simulink model "HydroEye_6DOF_SITL"  (R2024b)
settings: Solver=VariableStepAuto  StartTime=0.0  StopTime=1200  RelTol=1e-3
values from neighbouring files (symbols this model uses):
  b = 2    [HydroEye.m]
  c = 0.35    [HydroEye.m]
  CD = reshape(AeroLong.CD,length(alpha),length(elevator))    [HydroEye.m]
  cg = [0.5808 0 0.01]    [HydroEye.m]
  CL = reshape(AeroLong.CL,length(alpha),length(elevator))    [HydroEye.m]
  Cl = reshape(AeroLat.Cl,length(beta),length(rudder))    [HydroEye.m]
  Clp = -0.46415*pi/180    (= -0.00810094572313)    [HydroEye.m]
  Clr = 0.12437*pi/180    (= 0.00217066599071)    [HydroEye.m]
  Cm = reshape(AeroLong.Cm,length(alpha),length(elevator))    [HydroEye.m]
  Cmq = -5.4623*pi/180    (= -0.0953351197317)    [HydroEye.m]
  Cn = reshape(AeroLat.Cn,length(beta),length(rudder))    [HydroEye.m]
  Cnp = -0.05958*pi/180    (= -0.00103986716834)    [HydroEye.m]
  Cnr = -0.03820*pi/180    (= -0.000666715774262)    [HydroEye.m]
  cp = [0.519 0 -0018]    [HydroEye.m]
  current = [11.43 13.89 16.79 20.26 	25.87 31.71 37.21 44.10	]    [HydroEye.m]
  CY = reshape(AeroLat.CY,length(beta),length(rudder))    [HydroEye.m]
  mass = 7    [HydroEye.m]
  thrust = [1798 2069 2380 2771 3241 3738 4145 4635]/1000    [HydroEye.m]
undefined symbols (not defined in the file or in its folder): alpha_vec_Cn0, b_ref, beta_vec_Cn0, Clbeta, Clda, Cm0, Cmda, Cmde, Cn0, Cnda, CX0, CXda, CXde, CYbeta, CYda, CZ0, CZda, CZde, d_ref, Earth, F, Light, MIL, WGS84
libraries: simulink_extras x6, slpidlib x6, aerolibwind2 x3, aerolibasang x2, shared6dof x1, aerolibatmos2 x1, aerolibadyn x1, aerolibtransform2 x1
(part 2 of 2)

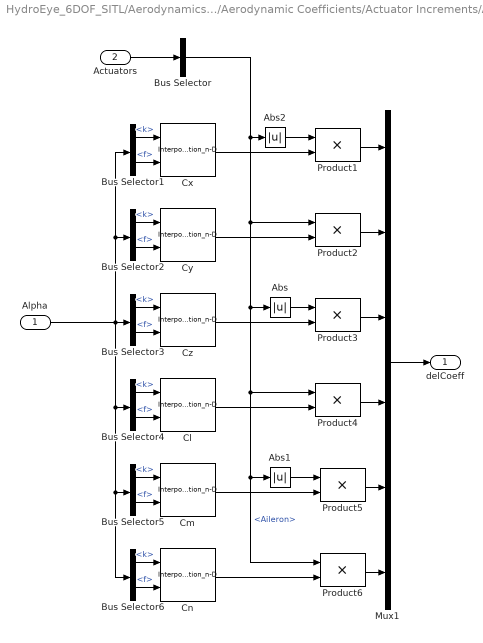
== system HydroEye_6DOF_SITL/Aerodynamics/Aerodynamic Coefficients/Actuator Increments/Ailerons ==
  Alpha : Inport
  Actuators : Inport  Port=2
  Abs : Abs
  Abs1 : Abs
  Abs2 : Abs
  Bus Selector : BusSelector  OutputSignals=Aileron
  Bus Selector{1..6} (6 alike) : BusSelector  OutputSignals=k,f
  Cl : Interpolation_n-D  NumberOfTableDimensions=1  Table=Clda  RemoveProtectionIndex=on
      settings: InputPortMap=u0,u1
  Cm : Interpolation_n-D  NumberOfTableDimensions=1  Table=Cmda  RemoveProtectionIndex=on
      settings: InputPortMap=u0,u1
  Cn : Interpolation_n-D  NumberOfTableDimensions=1  Table=Cnda  RemoveProtectionIndex=on
      settings: InputPortMap=u0,u1
  Cx : Interpolation_n-D  NumberOfTableDimensions=1  Table=CXda  RemoveProtectionIndex=on
      settings: InputPortMap=u0,u1
  Cy : Interpolation_n-D  NumberOfTableDimensions=1  Table=CYda  RemoveProtectionIndex=on
      settings: InputPortMap=u0,u1
  Cz : Interpolation_n-D  NumberOfTableDimensions=1  Table=CZda  RemoveProtectionIndex=on
      settings: InputPortMap=u0,u1
  Mux1 : Mux  Inputs=6
  Product{1..6} (6 alike) : Product  InputSameDT=on  SaturateOnIntegerOverflow=on  OutDataTypeStr=Inherit: Same as first input
  delCoeff : Outport  VectorParamsAs1DForOutWhenUnconnected=off
  wires:
  Actuators/1 -> Bus Selector/1
  Mux1/1 -> delCoeff/1
  Product1/1 -> Mux1/1
  Cx/1 -> Product1/2
  Product2/1 -> Mux1/2
  Cy/1 -> Product2/2
  Product3/1 -> Mux1/3
  Cz/1 -> Product3/2
  Cl/1 -> Product4/2
  Product4/1 -> Mux1/4
  Cm/1 -> Product5/2
  Product5/1 -> Mux1/5
  Cn/1 -> Product6/2
  Product6/1 -> Mux1/6
  Bus Selector/1 -> Product6/1, Abs1/1, Product4/1, Abs/1, Product2/1, Abs2/1  "<Aileron>"
  Abs/1 -> Product3/1
  Abs1/1 -> Product5/1
  Abs2/1 -> Product1/1
  Alpha/1 -> Bus Selector1/1, Bus Selector2/1, Bus Selector5/1, Bus Selector6/1, Bus Selector4/1, Bus Selector3/1
  Bus Selector1/1 -> Cx/1  "<k>"
  Bus Selector1/2 -> Cx/2  "<f>"
  Bus Selector2/1 -> Cy/1  "<k>"
  Bus Selector2/2 -> Cy/2  "<f>"
  Bus Selector3/1 -> Cz/1  "<k>"
  Bus Selector3/2 -> Cz/2  "<f>"
  Bus Selector4/1 -> Cl/1  "<k>"
  Bus Selector4/2 -> Cl/2  "<f>"
  Bus Selector5/1 -> Cm/1  "<k>"
  Bus Selector5/2 -> Cm/2  "<f>"
  Bus Selector6/1 -> Cn/1  "<k>"
  Bus Selector6/2 -> Cn/2  "<f>"

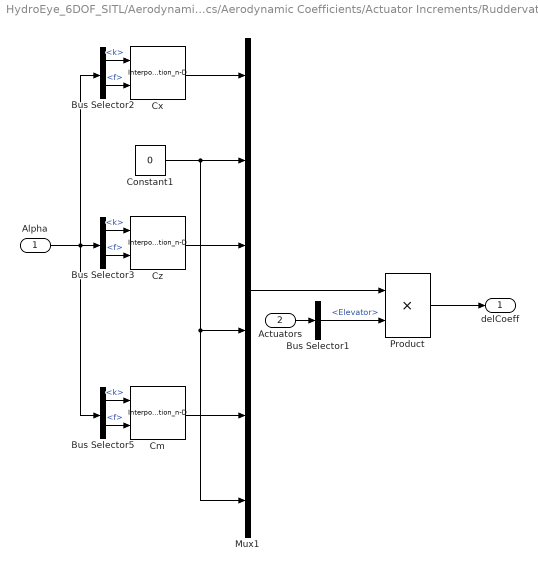
== system HydroEye_6DOF_SITL/Aerodynamics/Aerodynamic Coefficients/Actuator Increments/Ruddervators ==
  Alpha : Inport
  Actuators : Inport  Port=2
  Bus Selector1 : BusSelector  OutputSignals=Elevator
  Bus Selector2 : BusSelector  OutputSignals=k,f
  Bus Selector3 : BusSelector  OutputSignals=k,f
  Bus Selector5 : BusSelector  OutputSignals=k,f
  Cm : Interpolation_n-D  NumberOfTableDimensions=1  Table=Cmde  RemoveProtectionIndex=on
      settings: InputPortMap=u0,u1
  Constant1 : Constant  Value=0
  Cx : Interpolation_n-D  NumberOfTableDimensions=1  Table=CXde  RemoveProtectionIndex=on
      settings: InputPortMap=u0,u1
  Cz : Interpolation_n-D  NumberOfTableDimensions=1  Table=CZde  RemoveProtectionIndex=on
      settings: InputPortMap=u0,u1
  Mux1 : Mux  Inputs=6
  Product : Product  InputSameDT=on  SaturateOnIntegerOverflow=on  OutDataTypeStr=Inherit: Same as first input
  delCoeff : Outport  VectorParamsAs1DForOutWhenUnconnected=off
  wires:
  Product/1 -> delCoeff/1
  Mux1/1 -> Product/1
  Alpha/1 -> Bus Selector2/1, Bus Selector3/1, Bus Selector5/1
  Cx/1 -> Mux1/1
  Cz/1 -> Mux1/3
  Cm/1 -> Mux1/5
  Constant1/1 -> Mux1/2, Mux1/4, Mux1/6
  Actuators/1 -> Bus Selector1/1
  Bus Selector1/1 -> Product/2  "<Elevator>"
  Bus Selector2/1 -> Cx/1  "<k>"
  Bus Selector2/2 -> Cx/2  "<f>"
  Bus Selector3/1 -> Cz/1  "<k>"
  Bus Selector3/2 -> Cz/2  "<f>"
  Bus Selector5/1 -> Cm/1  "<k>"
  Bus Selector5/2 -> Cm/2  "<f>"

== system HydroEye_6DOF_SITL/Aerodynamics/Aerodynamic Coefficients/Body Rate Damping/p ==
  Alpha : Inport
  Bus Selector : BusSelector  OutputSignals=k,f
  Bus Selector1 : BusSelector  OutputSignals=k,f
  Cl : Interpolation_n-D  NumberOfTableDimensions=1  Table=Clp  RemoveProtectionIndex=on
      settings: InputPortMap=u0,u1
  Cn : Interpolation_n-D  NumberOfTableDimensions=1  Table=Cnp  RemoveProtectionIndex=on
      settings: InputPortMap=u0,u1
  Constant1 : Constant  Value=0
  Mux1 : Mux  Inputs=6
  delCoeff : Outport  VectorParamsAs1DForOutWhenUnconnected=off
  wires:
  Mux1/1 -> delCoeff/1
  Constant1/1 -> Mux1/1, Mux1/5, Mux1/3, Mux1/2  "Cxp"
  Cn/1 -> Mux1/6
  Cl/1 -> Mux1/4  "Cl"
  Alpha/1 -> Bus Selector/1, Bus Selector1/1
  Bus Selector/1 -> Cl/1  "<k>"
  Bus Selector/2 -> Cl/2  "<f>"
  Bus Selector1/1 -> Cn/1  "<k>"
  Bus Selector1/2 -> Cn/2  "<f>"

== system HydroEye_6DOF_SITL/Aerodynamics/Aerodynamic Coefficients/Body Rate Damping/q ==
  Alpha : Inport
  Bus Selector1 : BusSelector  OutputSignals=k,f
  Cmq : Interpolation_n-D  NumberOfTableDimensions=1  Table=Cmq  RemoveProtectionIndex=on
      settings: InputPortMap=u0,u1
  Constant3 : Constant  Value=0
  Mux1 : Mux  Inputs=6
  delCoeff : Outport  VectorParamsAs1DForOutWhenUnconnected=off
  wires:
  Cmq/1 -> Mux1/5
  Constant3/1 -> Mux1/1, Mux1/2, Mux1/3, Mux1/6, Mux1/4
  Mux1/1 -> delCoeff/1
  Alpha/1 -> Bus Selector1/1
  Bus Selector1/1 -> Cmq/1  "<k>"
  Bus Selector1/2 -> Cmq/2  "<f>"

== system HydroEye_6DOF_SITL/Aerodynamics/Aerodynamic Coefficients/Body Rate Damping/r ==
  Alpha : Inport
  Bus Selector : BusSelector  OutputSignals=k,f
  Bus Selector1 : BusSelector  OutputSignals=k,f
  Cl : Interpolation_n-D  NumberOfTableDimensions=1  Table=Clr  RemoveProtectionIndex=on
      settings: InputPortMap=u0,u1
  Cn : Interpolation_n-D  NumberOfTableDimensions=1  Table=Cnr  RemoveProtectionIndex=on
      settings: InputPortMap=u0,u1
  Constant : Constant  Value=0
  Mux1 : Mux  Inputs=6
  delCoeff : Outport  VectorParamsAs1DForOutWhenUnconnected=off
  wires:
  Cn/1 -> Mux1/6
  Cl/1 -> Mux1/4  "Cl"
  Constant/1 -> Mux1/1, Mux1/2, Mux1/5, Mux1/3  "Cxr"
  Mux1/1 -> delCoeff/1
  Alpha/1 -> Bus Selector1/1, Bus Selector/1
  Bus Selector/1 -> Cl/1  "<k>"
  Bus Selector/2 -> Cl/2  "<f>"
  Bus Selector1/1 -> Cn/1  "<k>"
  Bus Selector1/2 -> Cn/2  "<f>"
